simulink model "frequencyLQR"  (R2024a)
settings: Solver=ode1be  StartTime=0.0  StopTime=inf  FixedStep=0.1  RelTol=1e-6  EnableMultiTasking=on
values from neighbouring files (symbols this model uses):
  d = data(data.u_max==u_max & data.u_step==u_steps(j),:)    [writeBlockResponse.m]
  u_bar = (2*0.00283*9.81/(1.225*4*3.14*0.02^2*0.47*par_ODE(1)^2))^(1/(2*par_ODE(2)))    [systemIdentification.m]
undefined symbols (not defined in the file or in its folder): a, b, c, L, ln
libraries: arduinolib x2
settings Model: ExtModeTrigDuration=2  Creator=twallema  LastModifiedBy=twallema
settings SolverCC: AlgebraicLoopSolver=TrustRegion
settings OptimizationCC: EnhancedBackFolding=on  PassReuseOutputArgsThreshold=0  MaxStackSize=64  OptimizeBlockOrder=speed  DifferentSizesBufferReuse=on  OptimizationCustomize=off
settings DebuggingCC: ParameterTunabilityLossMsg=error  UnconnectedInputMsg=warning  UnconnectedOutputMsg=warning  UnconnectedLineMsg=warning
settings HardwareCC: ProdBitPerInt=16  ProdBitPerPointer=16  ProdBitPerSizeT=16  ProdBitPerPtrDiffT=16  ProdLargestAtomicFloat=None  ProdWordSize=8  ProdHWDeviceType=Atmel->AVR  UseEmbeddedCoderFeatures=off  UseSimulinkCoderFeatures=off
settings ModelReferenceCC: EnableRefExpFcnMdlSchedulingChecks=on
settings SFSimCC: MATLABDynamicMemAlloc=off  CustomCodeUndefinedFunction=UseInterfaceOnly
settings RTWCC: Description=Embedded Coder  SystemTargetFile=ert.tlc  HardwareBoard=Arduino Uno  TemplateMakefile=ert_default_tmf  GenerateReport=on  Toolchain=Arduino AVR  BuildConfiguration=Faster Runs  LaunchReport=on  GPUComputeCapability=3.5  DLArmComputeVersion=19.05
settings CodeAppCC: ForceParamTrailComments=on  OperatorAnnotations=on
settings ERTTargetCC: ERTCustomFileBanners=off  SupportContinuousTime=on  SupportNonInlinedSFcns=on  RemoveResetFunc=off  SupportVariableSizeSignals=on  ModelStepFunctionPrototypeControlCompliant=off  ExtModeStaticAllocSize=250

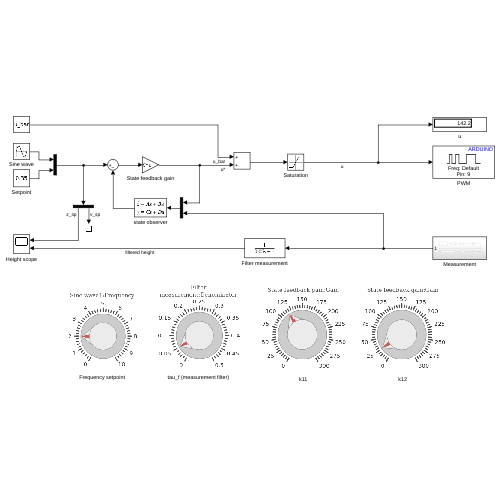
[thumbnail: Simulink's stored preview of the top-level diagram]
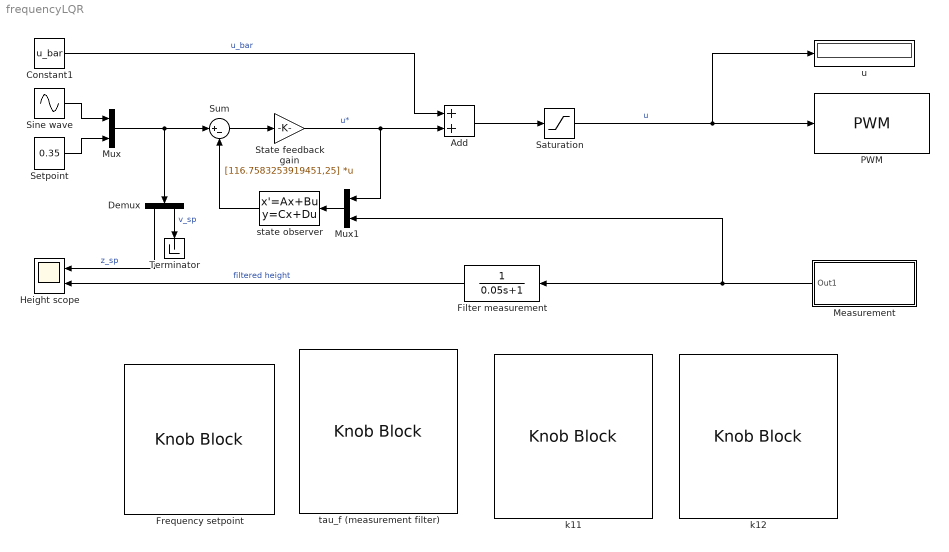
== system frequencyLQR ==
  Add : Sum
  Constant1 : Constant  Value=u_bar
  Demux : Demux  Outputs=2
  Filter measurement : TransferFcn  Denominator=[0.05,1]
  Frequency setpoint : KnobBlock  ScaleMax=10  TickInterval=1
  Height scope : Scope  NumInputPorts=2
  Measurement : Subsystem
  Mux : Mux  Inputs=2
  Mux1 : Mux  Inputs=2
  PWM : arduinolib/PWM  pinNumber=9  frequencyType=Default  desiredFrequency=490.2  achievableFrequency=490.2
  Saturation : Saturate  UpperLimit=255  LowerLimit=0
  Setpoint : Constant  Value=0.35
  Sine wave : Sin  Amplitude=0.1  Bias=0.35  Frequency=1.950676781221606  SampleTime=0
  State feedback gain : Gain  Gain=[116.7583253919451,25]  Multiplication=Matrix(K*u)
  Sum : Sum  Inputs=|+-
  Terminator : Terminator
  k11 : KnobBlock  ScaleMax=300
  k12 : KnobBlock  ScaleMax=300
  state observer : StateSpace  A=(a-L*c)  B=[b-L*d L]  C=eye(2)  D=[0, 0; 0, 0]  InitialCondition=[0; 0]
  tau_f (measurement filter) : KnobBlock  ScaleMax=0.5
  u : Display
  wires:
  Saturation/1 -> PWM/1, u/1  "u"
  Sum/1 -> State feedback gain/1
  State feedback gain/1 -> Mux1/1, Add/2  "u*"
  Constant1/1 -> Add/1  "u_bar"
  Add/1 -> Saturation/1
  Demux/2 -> Terminator/1  "v_sp"
  Demux/1 -> Height scope/1  "z_sp"
  state observer/1 -> Sum/2
  Mux1/1 -> state observer/1
  Measurement/1(Out1) -> Mux1/2, Filter measurement/1
  Filter measurement/1 -> Height scope/2  "filtered height"
  Sine wave/1 -> Mux/1
  Setpoint/1 -> Mux/2
  Mux/1 -> Sum/1, Demux/1

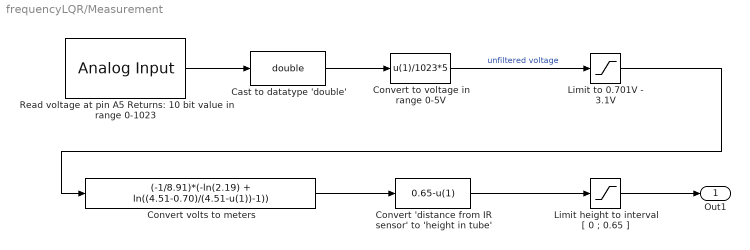
== system frequencyLQR/Measurement ==
  Cast to datatype 'double' : DataTypeConversion  OutDataTypeStr=double  SaturateOnIntegerOverflow=off  RndMeth=Floor
  Convert 'distance from IR sensor' to 'height in tube' : Fcn  Expr=0.65-u(1)
  Convert to voltage in range 0-5V : Fcn  Expr=u(1)/1023*5
  Convert volts to meters : Fcn  Expr=(-1/8.91)*(-ln(2.19) + ln((4.51-0.70)/(4.51-u(1))-1))
  Limit height to interval [ 0 ; 0.65 ] : Saturate  UpperLimit=0.65  LowerLimit=0
  Limit to 0.701V - 3.1V : Saturate  UpperLimit=3.1  LowerLimit=0.701
  Read voltage at pin A5 Returns: 10 bit value in range 0-1023 : arduinolib/Analog Input  pinNumber=5  ReadResultsOnly=off  ConversionTriggerSource=Software  ExternalTriggerType=uint32(0)  OutputDataType=uint16  EnableConversionCompleteNotify=off  EnableOuputStatus=off  SampleTime=0.1  blockPlatform=arduino
  Out1 : Outport  VectorParamsAs1DForOutWhenUnconnected=off
  wires:
  Convert 'distance from IR sensor' to 'height in tube'/1 -> Limit height to interval [ 0 ; 0.65 ]/1
  Cast to datatype 'double'/1 -> Convert to voltage in range 0-5V/1
  Read voltage at pin A5 Returns: 10 bit value in range 0-1023/1 -> Cast to datatype 'double'/1
  Limit height to interval [ 0 ; 0.65 ]/1 -> Out1/1
  Convert volts to meters/1 -> Convert 'distance from IR sensor' to 'height in tube'/1
  Limit to 0.701V - 3.1V/1 -> Convert volts to meters/1
  Convert to voltage in range 0-5V/1 -> Limit to 0.701V - 3.1V/1  "unfiltered voltage"
